simulink model "admire_sim_NDI"  (Simulink 8.4)
settings: Solver=ode4  SolverMode=SingleTasking  StartTime=0.0  StopTime=1000  FixedStep=dt  RelTol=1e-3  AbsTol=1e-6
InitFcn:
  | INIT_NDI
StartFcn:
  | tic
StopFcn:
  | toctime=toc;
  | fprintf('Actual Time = %g\nSim Time = %g\n',toctime,tout(end))
  | % Make plots
  | %admire_sim_plot
  | figure
  | plot3(yout(:,11),yout(:,10),-yout(:,12),'*-');grid
  | xlabel('East (m)');ylabel('North (m)');zlabel('Alt (m)')
  | view([0 0 1])
  | hold on
  | plot3(Ywpt,Xwpt,0*Xwpt,'r^-','MarkerSize',10)
  | axis equal
  | hold off
values from neighbouring files (symbols this model uses):
  a1 = (180*d2r)/(80^3)    (= 6.13592315154e-06)    [INIT_LINEAR.m]    (also in INIT_NDI.m)
  a2 = (24*d2r)/(80^3)    (= 8.18123086872e-07)    [INIT_LINEAR.m]    (also in INIT_NDI.m)
  Abare = [-0.0369710265542 -0.00338320638614 0 0 0.00101076287488 0 0 0 0 1.00000000002 0 1.7763568394e-12 ... (784 elements, 28x28)]    [Trim_M0p22ALT20_LinDATA.mat]    (also in Trim_M0p3ALT2000_LinDATA.mat = [-0.0208061645292 -0.00191640084378 0 0 0.000610808752105 0 )
  Altcmd_t = [ 0    1   100 200  300  425  450  550  600  700  800  880  980]    [INIT_NDI.m]
  Altcmd_v = [20  20   20   1500 1500 1500 1500 3000 3000 4000 4000 6000 6000]    [INIT_NDI.m]
  Bbare = [-1.10043807057 0.00182125944543 -0.00701366565749 0.707306131876 1.12037014439 -0.330899025785 0 0 0 0 0 0 ... (448 elements, 28x16)]    [Trim_M0p22ALT20_LinDATA.mat]    (also in Trim_M0p3ALT2000_LinDATA.mat = [-1.42042676365 -0.000549876720984 -0.00633411409606 0.84954)
  bref = 10    [INIT_NDI.m]
  C1 = ((Iy-Iz)*Iz-Ixz^2)/GG    (= -0.958151081688)    [INIT_NDI.m]
  C2 = (Ix-Iy+Iz)*Ixz/GG    (= 0.0484690861804)    [INIT_NDI.m]
  C3 = Iz/GG    (= 4.77597824802e-05)    [INIT_NDI.m]
  C4 = Ixz/GG    (= 1.18217283367e-06)    [INIT_NDI.m]
  C5 = (Iz-Ix)/Iy    (= 0.987654320988)    [INIT_NDI.m]
  C6 = Ixz/Iy    (= 0.0308641975309)    [INIT_NDI.m]
  C7 = 1/Iy    (= 1.23456790123e-05)    [INIT_NDI.m]
  C8 = (Ix*(Ix-Iy)+Ixz^2)/GG    (= -0.592859676085)    [INIT_NDI.m]
  C9 = Ix/GG    (= 9.93025180281e-06)    [INIT_NDI.m]
  CAmethod = 1    [ACA_init.m]    (also in INIT_LINEAR.m = 0; INIT_NDI.m = 0)
  Canard_max = interp1(M_vec,[25 25 25 15 15 15 15 15]*d2r,Mach,'next')    [INIT_LINEAR.m]    (also in INIT_NDI.m = [25 25 25 15 15 15 15 15]*d2r)
  Canard_min = interp1(M_vec,[-55 -55 -25 -15 -15 -15 -15 -15]*d2r,Mach,'next')    [INIT_LINEAR.m]    (also in INIT_NDI.m = [-55 -55 -25 -15 -15 -15 -15 -15]*d2r)
  CB = zeros(3,NumU)    [ACA_init.m]    (also in INIT_NDI.m = CCV*Bbare)
  CC = [C3 0 C4;0 C7 0;C4 0 C9]    [INIT_NDI.m]
  CCV = [CCV zeros(3,22)]    [INIT_LINEAR.m]    (also in INIT_NDI.m)
  cref = 5.2    [INIT_NDI.m]
  d2r = pi/180    (= 0.0174532925199)    [ACA_init.m]    (also in INIT_LINEAR.m; INIT_NDI.m)
  dalpha_err = 0    [Trim_M0p22ALT20_LinDATA.mat]    (also in Trim_M0p3ALT2000_LinDATA.mat)
  dalt_err = 0    [Trim_M0p22ALT20_LinDATA.mat]    (also in Trim_M0p3ALT2000_LinDATA.mat)
  dbeta_err = 0    [Trim_M0p22ALT20_LinDATA.mat]    (also in Trim_M0p3ALT2000_LinDATA.mat)
  ddc_bw = 0    [Trim_M0p22ALT20_LinDATA.mat]    (also in Trim_M0p3ALT2000_LinDATA.mat)
  ddc_rate = 0    [Trim_M0p22ALT20_LinDATA.mat]    (also in Trim_M0p3ALT2000_LinDATA.mat)
  ddei_bw = 0    [Trim_M0p22ALT20_LinDATA.mat]    (also in Trim_M0p3ALT2000_LinDATA.mat)
  ddei_rate = 0    [Trim_M0p22ALT20_LinDATA.mat]    (also in Trim_M0p3ALT2000_LinDATA.mat)
  ddey_bw = 0    [Trim_M0p22ALT20_LinDATA.mat]    (also in Trim_M0p3ALT2000_LinDATA.mat)
  ddey_rate = 0    [Trim_M0p22ALT20_LinDATA.mat]    (also in Trim_M0p3ALT2000_LinDATA.mat)
  ddle_bw = 0    [Trim_M0p22ALT20_LinDATA.mat]    (also in Trim_M0p3ALT2000_LinDATA.mat)
  ddle_rate = 0    [Trim_M0p22ALT20_LinDATA.mat]    (also in Trim_M0p3ALT2000_LinDATA.mat)
  ddr_bw = 0    [Trim_M0p22ALT20_LinDATA.mat]    (also in Trim_M0p3ALT2000_LinDATA.mat)
  ddr_rate = 0    [Trim_M0p22ALT20_LinDATA.mat]    (also in Trim_M0p3ALT2000_LinDATA.mat)
  dt = 0.01    [ACA_init.m]    (also in INIT_LINEAR.m; INIT_NDI.m)
  DTY_max = 0.002    [ACA_init.m]    (also in INIT_LINEAR.m; INIT_NDI.m)
  DTY_min = -0.002    [ACA_init.m]    (also in INIT_LINEAR.m; INIT_NDI.m)
  DTZ_max = 0.002    [ACA_init.m]    (also in INIT_LINEAR.m; INIT_NDI.m)
  DTZ_min = -0.002    [ACA_init.m]    (also in INIT_LINEAR.m; INIT_NDI.m)
  du = [eye(7,7)*d2r eye(7,7)*(-d2r);zeros(20,14)]    [INIT_NDI.m]
  dVt_err = 0    [Trim_M0p22ALT20_LinDATA.mat]    (also in Trim_M0p3ALT2000_LinDATA.mat)
  dx0bare = [-0.418180446269 0.000900932997672 0 0 -2.2213523116e-08 0 0 0 0 74.8477877145 0 0]    [Trim_M0p22ALT20_LinDATA.mat]    (also in Trim_M0p3ALT2000_LinDATA.mat = [-0.342751146187 0.000400431081223 0 0 -4.49007756074e-09 0 )
  Elevon_max = interp1(M_vec,[30 30 25 25 25 25 25 25]*d2r,Mach,'next')    [INIT_LINEAR.m]    (also in INIT_NDI.m = [30 30 25 25 25 25 25 25]*d2r)
  Elevon_min = interp1(M_vec,[-30 -30 -30 -30 -30 -30 -30 -30]*d2r,Mach,'next')    [INIT_LINEAR.m]    (also in INIT_NDI.m = [-30 -30 -30 -30 -30 -30 -30 -30]*d2r)
  G = [ 0 1 0 ... (first row only)    [ACA_init.m]    (also in INIT_LINEAR.m = [ 1 0 0; INIT_NDI.m)
  kcb = 2.5    [INIT_NDI.m]
  kfb = -0.4    [INIT_NDI.m]
  kib = 0.2    [INIT_NDI.m]
  kpb = 0.8    [INIT_NDI.m]
  LEF_max = interp1(M_vec,[30 30 30 20 20 15 10 10]*d2r,Mach,'next')    [INIT_LINEAR.m]    (also in INIT_NDI.m = [30 30 30 20 20 15 10 10]*d2r)
  LEF_min = interp1(M_vec,[-10 -10 -10 -10 -10 -10 -10 -10]*d2r,Mach,'next')    [INIT_LINEAR.m]    (also in INIT_NDI.m = [-10 -10 -10 -10 -10 -10 -10 -10]*d2r)
  LG_max = 1    [ACA_init.m]    (also in INIT_LINEAR.m; INIT_NDI.m)
  LG_min = 0    [ACA_init.m]    (also in INIT_LINEAR.m; INIT_NDI.m)
  LPmethod = 3    [ACA_init.m]    (also in INIT_LINEAR.m = 0; INIT_NDI.m = 0; LPwrap.m = 0; LPwrap_1.m = 0)
  M_vec = [0 0 0]    [DAwrap.m]    (also in INIT_LINEAR.m = [0 0.5 0.8 0.9 0.95 1.4 1.5 2.5]; INIT_NDI.m = [0 0.5 0.8 0.9 0.95 1.4 1.5 2.5])
  mass = 9100    [INIT_NDI.m]
  NumU = 16    [ACA_init.m]    (also in INIT_LINEAR.m; INIT_NDI.m; test.m; test_LPwrap.m)
  nwpt = 5    [INIT_NDI.m]
  PD_max = 10    [ACA_init.m]    (also in INIT_LINEAR.m; INIT_NDI.m)
  PD_min = -10    [ACA_init.m]    (also in INIT_LINEAR.m; INIT_NDI.m)
  PHIcmd_t = [0 1 1+dt 30 30+dt 60 60+dt 90 90+dt 120 120+dt 150 150+dt 180 180+dt 210 210+dt 240 240+dt 270 270+dt 300 300+dt 330 330+dt]    [INIT_NDI.m]
  PHIcmd_v = [0 0 15   15 -15   -15 0    0   30   30  -30    -30 0      0   45     45   0     0    -45   -45   0     0   -60   -60 0]    [INIT_NDI.m]
  Pmode = 3    [INIT_NDI.m]
  r2d = 180/pi    (= 57.2957795131)    [ACA_init.m]    (also in INIT_LINEAR.m; INIT_NDI.m)
  rlimit_c = 0.87260034904    [Trim_M0p22ALT20_LinDATA.mat]    (also in Trim_M0p3ALT2000_LinDATA.mat)
  rlimit_ie = 2.61780104712    [Trim_M0p22ALT20_LinDATA.mat]    (also in Trim_M0p3ALT2000_LinDATA.mat)
  rlimit_le = 0.174520069808    [Trim_M0p22ALT20_LinDATA.mat]    (also in Trim_M0p3ALT2000_LinDATA.mat)
  rlimit_oe = 2.61780104712    [Trim_M0p22ALT20_LinDATA.mat]    (also in Trim_M0p3ALT2000_LinDATA.mat)
  rlimit_r = 1.74520069808    [Trim_M0p22ALT20_LinDATA.mat]    (also in Trim_M0p3ALT2000_LinDATA.mat)
  Rmode = 3    [INIT_NDI.m]
  Rudder_max = interp1(M_vec,[30 30 25 20 15 15 15 10]*d2r,Mach,'next')    [INIT_LINEAR.m]    (also in INIT_NDI.m = [30 30 25 20 15 15 15 10]*d2r)
  Rudder_min = interp1(M_vec,[-30 -30 -25 -20 -15 -15 -15 -10]*d2r,Mach,'next')    [INIT_LINEAR.m]    (also in INIT_NDI.m = [-30 -30 -25 -20 -15 -15 -15 -10]*d2r)
  Sref = 45    [INIT_NDI.m]
  TSS_max = 1    [ACA_init.m]    (also in INIT_LINEAR.m; INIT_NDI.m)
  TSS_min = 0    [ACA_init.m]    (also in INIT_LINEAR.m; INIT_NDI.m)
  u0fcs = [0 74.8477877145 0 0 -0.0114511280235]    [Trim_M0p22ALT20_LinDATA.mat]    (also in Trim_M0p3ALT2000_LinDATA.mat = [0 99.7587452043 0 0 -0.00434812413209])
  u0new = [-0.00172441963734 -0.00172441963734 0.0557681770547 0.0557681770547 0.0557681770547 0.0557681770547 0 0 0 0.0785 0 0 ... (16 elements, 16x1)]    [Trim_M0p22ALT20_LinDATA.mat]    (also in Trim_M0p3ALT2000_LinDATA.mat = [-0.00056590748572 -0.00056590748572 0.0273345559009 0.02733)
  UD_max = 10    [ACA_init.m]    (also in INIT_LINEAR.m; INIT_NDI.m)
  UD_min = -10    [ACA_init.m]    (also in INIT_LINEAR.m; INIT_NDI.m)
  Upref = [0 0 0 0 0 0 0 0 0 0 0 0 0 0 0 0]'    [ACA_init.m]    (also in INIT_LINEAR.m; INIT_NDI.m)
  Upref_split = [[0 0 30 -30 -30 30 0]*d2r*.4 0 0 0 0 0 0 0 0 0]'    [INIT_NDI.m]
  Urlim = [350*d2r ... (first row only)    [ACA_init.m]    (also in INIT_NDI.m = [50*d2r)
  UseRL = 0    [ACA_init.m]    (also in INIT_NDI.m)
  Vcmd_t = [  0    1   100  200  300  425  450  550  600  700  800  880  980]    [INIT_NDI.m]
  Vcmd_v = Mcmd_v.*a    [INIT_NDI.m]
  VD_max = 10    [ACA_init.m]    (also in INIT_LINEAR.m; INIT_NDI.m)
  VD_min = -10    [ACA_init.m]    (also in INIT_LINEAR.m; INIT_NDI.m)
  WD_max = 10    [ACA_init.m]    (also in INIT_LINEAR.m; INIT_NDI.m)
  WD_min = -10    [ACA_init.m]    (also in INIT_LINEAR.m; INIT_NDI.m)
  Wp = W'*W    [ACA_init.m]    (also in INIT_LINEAR.m; INIT_NDI.m; test.m; test_LPwrap.m)
  Wpts = [0 1 2 3 4]    [INIT_NDI.m]
  x0 = [ max(eyp,zeros(n,1));max(-eyp,zeros(n,1));zeros(2*m,1)]    [LPwrap.m]    (also in LPwrap_1.m; LPwrap_par.m; Trim_M0p22ALT20_LinDATA.mat = [-8.62209818672e-05 -8.62209818672e-05 0.00278840885273 0.00; Trim_M0p3ALT2000_LinDATA.mat = [-2.8295374286e-05 -2.8295374286e-05 0.00136672779504 0.0013)
  x0bare = [74.8477877145 0.159877852888 0 0 0 0 0 0.159877852888 0 0 0 -20]    [Trim_M0p22ALT20_LinDATA.mat]    (also in Trim_M0p3ALT2000_LinDATA.mat = [99.7587452043 0.116024082006 0 0 0 0 0 0.116024082006 0 0 0)
  Xwpt = [0 4000 4000 0 0]*8    [INIT_NDI.m]
  y0bare = [74.8477877145 0.159877852888 0 0 0 0 0 0.159877852888 0 0 0 -20 ... (73 elements, 73x1)]    [Trim_M0p22ALT20_LinDATA.mat]    (also in Trim_M0p3ALT2000_LinDATA.mat = [99.7587452043 0.116024082006 0 0 0 0 0 0.116024082006 0 0 0)
  Ywpt = [0 0 4000 4000 0]*8    [INIT_NDI.m]
undefined symbols (not defined in the file or in its folder): CGIwrap, DAwrap, LPwrap, VJAwrap
libraries: simulink_extras x19, simulink x12
(part 2 of 5)

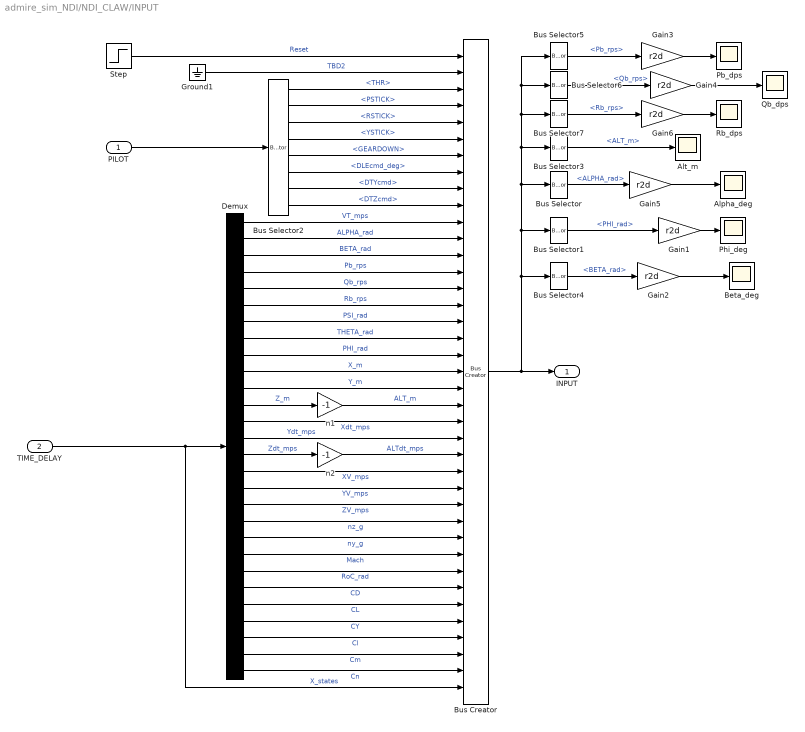
== system admire_sim_NDI/NDI_CLAW/INPUT ==
  PILOT : Inport
  TIME_DELAY : Inport  Port=2
  Alpha_deg : Scope
      settings: TimeRange=1000  YMin=0  YMax=16  SaveName=ScopeData9
  Alt_m : Scope
      settings: TimeRange=1000  YMin=0  YMax=7000  SaveName=ScopeData20
  Beta_deg : Scope
      settings: TimeRange=80  YMin=-10  YMax=15  SaveName=ScopeData32
  Bus Creator : BusCreator  Inputs=39
  Bus Selector : BusSelector  OutputSignals=ALPHA_rad
  Bus Selector1 : BusSelector  OutputSignals=PHI_rad
  Bus Selector2 : BusSelector  OutputSignals=THR,PSTICK,RSTICK,YSTICK,GEARDOWN,DLEcmd_deg,DTYcmd,DTZcmd
  Bus Selector3 : BusSelector  OutputSignals=ALT_m
  Bus Selector4 : BusSelector  OutputSignals=BETA_rad
  Bus Selector5 : BusSelector  OutputSignals=Pb_rps
  Bus Selector6 : BusSelector  OutputSignals=Qb_rps
  Bus Selector7 : BusSelector  OutputSignals=Rb_rps
  Demux : Demux  Outputs=28
  Gain{1..6} (6 alike) : Gain  Gain=r2d
  Ground1 : Ground
  Pb_dps : Scope
      settings: TimeRange=1000  YMin=-60  YMax=40  SaveName=ScopeData33
  Phi_deg : Scope
      settings: TimeRange=1000  YMin=-80  YMax=80  SaveName=ScopeData8
  Qb_dps : Scope
      settings: TimeRange=1000  YMax=10  SaveName=ScopeData34
  Rb_dps : Scope
      settings: TimeRange=80  YMin=16  YMax=22  SaveName=ScopeData35
  Step : Step  Time=dt  Before=1  After=0  SampleTime=dt
  n1 : Gain  Gain=-1
  n2 : Gain  Gain=-1
  INPUT : Outport
  wires:
  Bus Creator/1 -> INPUT/1, Bus Selector3/1, Bus Selector5/1, Bus Selector6/1, Bus Selector7/1, Bus Selector/1, Bus Selector1/1, Bus Selector4/1
  PILOT/1 -> Bus Selector2/1
  Bus Selector2/1 -> Bus Creator/3  "<THR>"
  Bus Selector2/2 -> Bus Creator/4  "<PSTICK>"
  Bus Selector2/3 -> Bus Creator/5  "<RSTICK>"
  Bus Selector2/4 -> Bus Creator/6  "<YSTICK>"
  Bus Selector2/5 -> Bus Creator/7  "<GEARDOWN>"
  Ground1/1 -> Bus Creator/2  "TBD2"
  Step/1 -> Bus Creator/1  "Reset"
  Bus Selector2/6 -> Bus Creator/8  "<DLEcmd_deg>"
  Bus Selector2/7 -> Bus Creator/9  "<DTYcmd>"
  Bus Selector2/8 -> Bus Creator/10  "<DTZcmd>"
  Demux/1 -> Bus Creator/11  "VT_mps"
  Demux/2 -> Bus Creator/12  "ALPHA_rad"
  Demux/5 -> Bus Creator/15  "Qb_rps"
  Demux/8 -> Bus Creator/18  "THETA_rad"
  Demux/3 -> Bus Creator/13  "BETA_rad"
  Demux/4 -> Bus Creator/14  "Pb_rps"
  Demux/6 -> Bus Creator/16  "Rb_rps"
  Demux/9 -> Bus Creator/19  "PHI_rad"
  Demux/10 -> Bus Creator/20  "X_m"
  Demux/11 -> Bus Creator/21  "Y_m"
  Demux/12 -> n1/1  "Z_m"
  n1/1 -> Bus Creator/22  "ALT_m"
  Demux/13 -> Bus Creator/23  "Xdt_mps"
  Demux/14 -> Bus Creator/24  "Ydt_mps"
  Demux/15 -> n2/1  "Zdt_mps"
  Demux/16 -> Bus Creator/26  "XV_mps"
  Demux/17 -> Bus Creator/27  "YV_mps"
  Demux/18 -> Bus Creator/28  "ZV_mps"
  Demux/19 -> Bus Creator/29  "nz_g"
  Demux/20 -> Bus Creator/30  "ny_g"
  Demux/21 -> Bus Creator/31  "Mach"
  Demux/22 -> Bus Creator/32  "RoC_rad"
  Demux/23 -> Bus Creator/33  "CD"
  Demux/24 -> Bus Creator/34  "CL"
  Demux/25 -> Bus Creator/35  "CY"
  Demux/26 -> Bus Creator/36  "Cl"
  Demux/27 -> Bus Creator/37  "Cm"
  Demux/28 -> Bus Creator/38  "Cn"
  Demux/7 -> Bus Creator/17  "PSI_rad"
  n2/1 -> Bus Creator/25  "ALTdt_mps"
  TIME_DELAY/1 -> Demux/1, Bus Creator/39  "X_states"
  Gain5/1 -> Alpha_deg/1
  Bus Selector/1 -> Gain5/1  "<ALPHA_rad>"
  Gain1/1 -> Phi_deg/1
  Bus Selector1/1 -> Gain1/1  "<PHI_rad>"
  Bus Selector3/1 -> Alt_m/1  "<ALT_m>"
  Gain2/1 -> Beta_deg/1
  Bus Selector4/1 -> Gain2/1  "<BETA_rad>"
  Bus Selector5/1 -> Gain3/1  "<Pb_rps>"
  Bus Selector6/1 -> Gain4/1  "<Qb_rps>"
  Bus Selector7/1 -> Gain6/1  "<Rb_rps>"
  Gain3/1 -> Pb_dps/1
  Gain4/1 -> Qb_dps/1
  Gain6/1 -> Rb_dps/1

== system admire_sim_NDI/NDI_CLAW/MissionManager ==
  INPUT : Inport
  ALT_table : Lookup  InputValues=Altcmd_t  Table=Altcmd_v  LookUpMeth=Interpolation-Use End Values
  Bus Creator : BusCreator  Inputs=8
  Bus Selector3 : BusSelector  OutputSignals=Xcmd,Xcmdm1,Ycmd,Ycmdm1,PHImax_rad
  Constant : Constant  Value=Vcmd_v(1)
  Constant1 : Constant  Value=Altcmd_v(1)
  Constant2 : Constant  Value=x0bare(1)
  Constant3 : Constant  Value=-x0bare(12)+50
  Constant4 : Constant  Value=-120
  Digital Clock : DigitalClock  SampleTime=dt
  Gain : Gain  Gain=0
  PHI_5 : Lookup  InputValues=PHIcmd_t  Table=PHIcmd_v  LookUpMeth=Interpolation-Use End Values
  Saturation : Saturate  UpperLimit=300  LowerLimit=0
  Sum : Sum  Inputs=|++
  V_table : Lookup  InputValues=Vcmd_t  Table=Vcmd_v  LookUpMeth=Interpolation-Use End Values
  WaypointNavigation : Subsystem
  MM : Outport
  wires:
  Digital Clock/1 -> Sum/1, V_table/1, ALT_table/1
  Bus Creator/1 -> MM/1
  PHI_5/1 -> Bus Creator/3  "PHIcmd_deg"
  INPUT/1 -> WaypointNavigation/1(INPUT)
  WaypointNavigation/1(WN) -> Bus Selector3/1
  Bus Selector3/1 -> Bus Creator/4  "<Xcmd>"
  Bus Selector3/2 -> Bus Creator/5  "<Xcmdm1>"
  Bus Selector3/3 -> Bus Creator/6  "<Ycmd>"
  Bus Selector3/4 -> Bus Creator/7  "<Ycmdm1>"
  Bus Selector3/5 -> Bus Creator/8  "<PHImax_rad>"
  V_table/1 -> Bus Creator/2  "Vcmd_mps"
  ALT_table/1 -> Bus Creator/1  "ALTcmd_m"
  Sum/1 -> Saturation/1
  Constant4/1 -> Sum/2
  Saturation/1 -> Gain/1
  Gain/1 -> PHI_5/1

== system admire_sim_NDI/NDI_CLAW/PILOT_Mod ==
  In1 : Inport
  Bus Creator1 : BusCreator  Inputs=9
  Bus Selector : BusSelector  OutputSignals=Fes_out,Vt_out,Fas_out,Frp_out,dle_out,ldg_out,dty_out,dtz_out,tss_out
  Gain1 : Gain  Gain=1/80
  Gain{2,5..9} (6 alike) : Gain
  Gain3 : Gain  Gain=1/80
  Gain4 : Gain  Gain=1/200
  PILOT : Outport
  wires:
  In1/1 -> Bus Selector/1
  Bus Selector/1 -> Gain1/1  "<Fes_out>"
  Bus Selector/2 -> Gain2/1  "<Vt_out>"
  Bus Selector/3 -> Gain3/1  "<Fas_out>"
  Bus Selector/4 -> Gain4/1  "<Frp_out>"
  Bus Selector/5 -> Gain5/1  "<dle_out>"
  Bus Selector/6 -> Gain6/1  "<ldg_out>"
  Bus Selector/7 -> Gain7/1  "<dty_out>"
  Bus Selector/8 -> Gain8/1  "<dtz_out>"
  Gain1/1 -> Bus Creator1/1  "PSTICK"
  Gain2/1 -> Bus Creator1/2  "Vcmd_mps"
  Gain3/1 -> Bus Creator1/3  "RSTICK"
  Gain4/1 -> Bus Creator1/4  "YSTICK"
  Gain5/1 -> Bus Creator1/5  "DLEcmd_deg"
  Gain6/1 -> Bus Creator1/6  "GEARDOWN"
  Gain7/1 -> Bus Creator1/7  "DTYcmd"
  Gain8/1 -> Bus Creator1/8  "DTZcmd"
  Gain9/1 -> Bus Creator1/9  "THR"
  Bus Creator1/1 -> PILOT/1
  Bus Selector/9 -> Gain9/1  "<tss_out>"

== system admire_sim_NDI/PILOT/Doublet ==
  Gain : Gain  Gain=.1
  Step : Step  SampleTime=0
  Step1 : Step  Time=1.1  After=-2  SampleTime=0
  Step2 : Step  Time=1.2  SampleTime=0
  Sum8 : Sum  Inputs=+++
  Out1 : Outport
  wires:
  Step/1 -> Sum8/1
  Step1/1 -> Sum8/2
  Step2/1 -> Sum8/3
  Sum8/1 -> Gain/1
  Gain/1 -> Out1/1

== system admire_sim_NDI/Aircraft response1/Sensor models/Subsystem To Gain-Scheduling ==
  note: Level III
  Vt [m/s] : Inport
  alt [m] : Inport  Port=2
  S-Function : S-Function  FunctionName=machno  EnableBusSupport=off
  Mach : Outport
  tag scope: Altitude=global, Mach=global
  wires:
  alt [m]/1 -> [Altitude], S-Function/2
  Vt [m/s]/1 -> S-Function/1
  S-Function/1 -> [Mach], Mach/1

== system admire_sim_NDI/NDI_CLAW/DynamicInversionControl/AERO_OBM ==
  INPUT : Inport
  uz : Inport  Port=2
  AeroLimits : Subsystem
  Bus Creator1 : BusCreator  Inputs=5
  Bus Selector : BusSelector  OutputSignals=Unom
  LinearOBM : Subsystem
  NonLinearOBM : Subsystem
  OBM : Outport
  wires:
  AeroLimits/1(Umin) -> Bus Creator1/4
  AeroLimits/2(Umax) -> Bus Creator1/5
  Bus Creator1/1 -> OBM/1
  uz/1 -> LinearOBM/2(uz), Bus Selector/1, NonLinearOBM/2(uz)
  Bus Selector/1 -> Bus Creator1/3  "<Unom>"
  INPUT/1 -> LinearOBM/1(INPUT), AeroLimits/1(Input), NonLinearOBM/1(INPUT)
  NonLinearOBM/1(CVdt_nom) -> Bus Creator1/1
  NonLinearOBM/2(CB) -> Bus Creator1/2

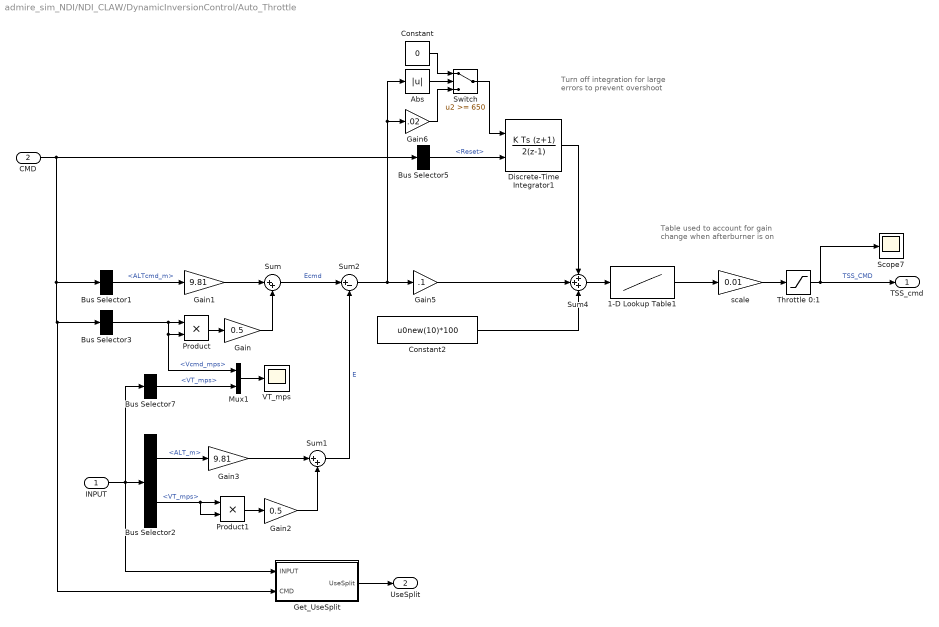
== system admire_sim_NDI/NDI_CLAW/DynamicInversionControl/Auto_Throttle ==
  note: Turn off integration for large
      | errors to prevent overshoot
  note: Table used to account for gain
      | change when afterburner is on
  INPUT : Inport
  CMD : Inport  Port=2
  1-D Lookup Table1 : Lookup_n-D  NumberOfTableDimensions=1  BreakpointsForDimension1=[0 80 300]  Table=[0 80 100]  ExtrapMethod=Clip  UseLastTableValue=on  RndMeth=Simplest  InputSameDT=on
  Abs : Abs
  Bus Selector1 : BusSelector  OutputSignals=ALTcmd_m
  Bus Selector2 : BusSelector  OutputSignals=ALT_m,VT_mps
  Bus Selector3 : BusSelector  OutputSignals=Vcmd_mps
  Bus Selector5 : BusSelector  OutputSignals=Reset
  Bus Selector7 : BusSelector  OutputSignals=VT_mps
  Constant : Constant  Value=0
  Constant2 : Constant  Value=u0new(10)*100
  Discrete-Time Integrator1 : DiscreteIntegrator  IntegratorMethod=Integration: Trapezoidal  ExternalReset=level  SampleTime=dt  LimitOutput=on  LowerSaturationLimit=-50
  Gain : Gain  Gain=0.5
  Gain1 : Gain  Gain=9.81
  Gain2 : Gain  Gain=0.5
  Gain3 : Gain  Gain=9.81
  Gain5 : Gain  Gain=.1
  Gain6 : Gain  Gain=.02
  Get_UseSplit : Subsystem
  Mux1 : Mux  Inputs=2
  Product : Product  RndMeth=Zero
  Product1 : Product  RndMeth=Zero
  Scope7 : Scope
      settings: TimeRange=20  YMin=0  YMax=1  SaveName=ScopeData11
  Sum : Sum  Inputs=|++
  Sum1 : Sum  Inputs=|++
  Sum2 : Sum  Inputs=|+-
  Sum4 : Sum  Inputs=+++
  Switch : Switch  Threshold=650
  Throttle 0:1 : Saturate  UpperLimit=TSS_max  LowerLimit=TSS_min  RndMeth=Ceiling
  VT_mps : Scope
      settings: TimeRange=1000  YMin=50  YMax=450  SaveName=ScopeData58
  scale : Gain  Gain=0.01
  TSS_cmd : Outport
  UseSplit : Outport  Port=2
  wires:
  CMD/1 -> Bus Selector1/1, Get_UseSplit/2(CMD), Bus Selector3/1, Bus Selector5/1
  Product/1 -> Gain/1
  Gain/1 -> Sum/2
  Product1/1 -> Gain2/1
  Bus Selector2/1 -> Gain3/1  "<ALT_m>"
  Gain2/1 -> Sum1/2
  Bus Selector2/2 -> Product1/1, Product1/2  "<VT_mps>"
  Sum/1 -> Sum2/1  "Ecmd"
  Sum1/1 -> Sum2/2  "E"
  Bus Selector5/1 -> Discrete-Time Integrator1/2  "<Reset>"
  Discrete-Time Integrator1/1 -> Sum4/1
  Sum2/1 -> Gain5/1, Gain6/1, Abs/1
  Bus Selector1/1 -> Gain1/1  "<ALTcmd_m>"
  Bus Selector3/1 -> Product/1, Product/2, Mux1/1  "<Vcmd_mps>"
  Sum4/1 -> 1-D Lookup Table1/1
  Abs/1 -> Switch/2
  Switch/1 -> Discrete-Time Integrator1/1
  Constant/1 -> Switch/1
  Gain6/1 -> Switch/3
  INPUT/1 -> Get_UseSplit/1(INPUT), Bus Selector7/1, Bus Selector2/1
  1-D Lookup Table1/1 -> scale/1
  Gain5/1 -> Sum4/2
  Mux1/1 -> VT_mps/1
  Bus Selector7/1 -> Mux1/2  "<VT_mps>"
  Get_UseSplit/1(UseSplit) -> UseSplit/1
  Constant2/1 -> Sum4/3
  scale/1 -> Throttle 0:1/1
  Throttle 0:1/1 -> TSS_cmd/1, Scope7/1  "TSS_CMD"
  Gain1/1 -> Sum/1
  Gain3/1 -> Sum1/1

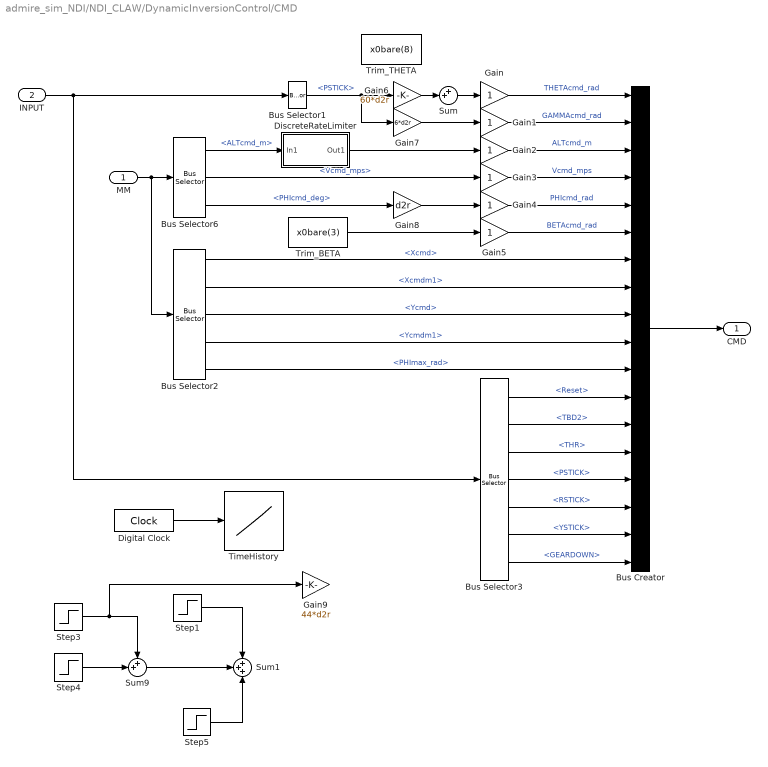
== system admire_sim_NDI/NDI_CLAW/DynamicInversionControl/CMD ==
  MM : Inport
  INPUT : Inport  Port=2
  Bus Creator : BusCreator  Inputs=18
  Bus Selector1 : BusSelector  OutputSignals=PSTICK
  Bus Selector2 : BusSelector  OutputSignals=Xcmd,Xcmdm1,Ycmd,Ycmdm1,PHImax_rad
  Bus Selector3 : BusSelector  OutputSignals=Reset,TBD2,THR,PSTICK,RSTICK,YSTICK,GEARDOWN
  Bus Selector6 : BusSelector  OutputSignals=ALTcmd_m,Vcmd_mps,PHIcmd_deg
  Digital Clock : DigitalClock  SampleTime=dt
  DiscreteRateLimiter : Subsystem
  Gain{,1..5} (6 alike) : Gain
  Gain6 : Gain  Gain=60*d2r
  Gain7 : Gain  Gain=6*d2r
  Gain8 : Gain  Gain=d2r
  Gain9 : Gain  Gain=44*d2r
  Step1 : Step  Time=70  SampleTime=dt
  Step3 : Step  Time=50  SampleTime=dt
  Step4 : Step  Time=60  After=-1  SampleTime=dt
  Step5 : Step  Time=60  After=-1  SampleTime=dt
  Sum : Sum  Inputs=++|
  Sum1 : Sum  Inputs=+++
  Sum9 : Sum  Inputs=++|
  TimeHistory : Lookup  InputValues=[0 20 30 40 50 60]  Table=[0 0 3 3 0 0]*d2r  LookUpMeth=Interpolation-Use End Values
  Trim_BETA : Constant  Value=x0bare(3)
  Trim_THETA : Constant  Value=x0bare(8)
  CMD : Outport
  wires:
  Bus Creator/1 -> CMD/1
  Gain/1 -> Bus Creator/1  "THETAcmd_rad"
  Gain1/1 -> Bus Creator/2  "GAMMAcmd_rad"
  Gain2/1 -> Bus Creator/3  "ALTcmd_m"
  Gain3/1 -> Bus Creator/4  "Vcmd_mps"
  Gain4/1 -> Bus Creator/5  "PHIcmd_rad"
  Gain5/1 -> Bus Creator/6  "BETAcmd_rad"
  Bus Selector1/1 -> Gain6/1, Gain7/1  "<PSTICK>"
  INPUT/1 -> Bus Selector1/1, Bus Selector3/1
  Gain7/1 -> Gain1/1
  Gain6/1 -> Sum/2
  Sum/1 -> Gain/1
  MM/1 -> Bus Selector6/1, Bus Selector2/1
  Bus Selector6/1 -> DiscreteRateLimiter/1(In1)  "<ALTcmd_m>"
  Bus Selector6/2 -> Gain3/1  "<Vcmd_mps>"
  Bus Selector6/3 -> Gain8/1  "<PHIcmd_deg>"
  Bus Selector2/1 -> Bus Creator/7  "<Xcmd>"
  Bus Selector2/2 -> Bus Creator/8  "<Xcmdm1>"
  Bus Selector2/3 -> Bus Creator/9  "<Ycmd>"
  Bus Selector2/4 -> Bus Creator/10  "<Ycmdm1>"
  Bus Selector2/5 -> Bus Creator/11  "<PHImax_rad>"
  Bus Selector3/1 -> Bus Creator/12  "<Reset>"
  Bus Selector3/2 -> Bus Creator/13  "<TBD2>"
  Bus Selector3/3 -> Bus Creator/14  "<THR>"
  Bus Selector3/4 -> Bus Creator/15  "<PSTICK>"
  Bus Selector3/5 -> Bus Creator/16  "<RSTICK>"
  Bus Selector3/6 -> Bus Creator/17  "<YSTICK>"
  Bus Selector3/7 -> Bus Creator/18  "<GEARDOWN>"
  Step3/1 -> Sum9/1, Gain9/1
  Step4/1 -> Sum9/2
  Sum9/1 -> Sum1/2
  Step1/1 -> Sum1/1
  Digital Clock/1 -> TimeHistory/1
  Step5/1 -> Sum1/3
  Trim_BETA/1 -> Gain5/1
  DiscreteRateLimiter/1(Out1) -> Gain2/1
  Gain8/1 -> Gain4/1

== system admire_sim_NDI/NDI_CLAW/DynamicInversionControl/ControlAllocation ==
  TSS_cmd : Inport
  UseSplit : Inport  Port=2
  CVdt_des : Inport  Port=3
  OBM : Inport  Port=4
  GetU : Subsystem
  PostProcess : Subsystem
  PreProcess : Subsystem
  Ucmd : Outport
  wires:
  PreProcess/1(PrePro) -> GetU/1(PrePro), PostProcess/2(PrePro)
  GetU/1(u) -> PostProcess/1(u)
  CVdt_des/1 -> PreProcess/1(CVdt_des)  "CVdt_des"
  OBM/1 -> PreProcess/2(OBM)
  UseSplit/1 -> PostProcess/3(UseSplit)
  PostProcess/1(Ucmd) -> Ucmd/1
  TSS_cmd/1 -> PostProcess/4(TSS_cmd)

== system admire_sim_NDI/NDI_CLAW/DynamicInversionControl/REG ==
  CMD : Inport
  INPUT : Inport  Port=2
  Mux : Mux  Inputs=3
  PitchReg : Subsystem
  RollReg : Subsystem
  YawReg : Subsystem
  CVdt_des : Outport
  wires:
  CMD/1 -> RollReg/1(CMD), YawReg/1(CMD), PitchReg/1(CMD)
  Mux/1 -> CVdt_des/1  "CVdt_des"
  PitchReg/1(MCVdt) -> Mux/2
  RollReg/1(LCVdt) -> Mux/1
  YawReg/1(NCVdt) -> Mux/3
  INPUT/1 -> RollReg/2(INPUT), PitchReg/2(INPUT), YawReg/2(INPUT)

== system admire_sim_NDI/NDI_CLAW/DynamicInversionControl/UcmdScope ==
  In1 : Inport
  Demux : Demux  Outputs=7
  Selector : Selector  InputPortWidth=16  Indices=[1:7]
  Ucmd_deg : Scope  NumInputPorts=7
      settings: TimeRange=1000  YMin=-10~-10~-10~-20~-20~-10~-4  YMax=10~10~20~10~10~20~4  SaveName=ScopeData51
  scale1 : Gain  Gain=r2d
  wires:
  Selector/1 -> scale1/1
  scale1/1 -> Demux/1
  In1/1 -> Selector/1
  Demux/2 -> Ucmd_deg/2  "LC_deg"
  Demux/1 -> Ucmd_deg/1  "RC_deg"
  Demux/5 -> Ucmd_deg/5  "LIE_deg"
  Demux/7 -> Ucmd_deg/7  "RUD_deg"
  Demux/6 -> Ucmd_deg/6  "LOE_deg"
  Demux/3 -> Ucmd_deg/3  "ROE_deg"
  Demux/4 -> Ucmd_deg/4  "RIE_deg"

== system admire_sim_NDI/NDI_CLAW/DynamicInversionControl/Unom ==
  Ucmd : Inport
  Bus Creator : BusCreator  Inputs=2
  Discrete-Time Integrator : DiscreteIntegrator  IntegratorMethod=Integration: Trapezoidal  InitialCondition=u0new  SampleTime=dt
  Get_Unom : Subsystem
  Sum2 : Sum  Inputs=|+-
  Unit Delay1 : UnitDelay  InitialCondition=u0new  SampleTime=dt
  Unit Delay2 : UnitDelay  InitialCondition=u0new  SampleTime=dt
  scale1 : Gain
  scale2 : Gain  Gain=20
  Upast : Outport
  wires:
  Discrete-Time Integrator/1 -> Unit Delay2/1, scale1/1
  Unit Delay1/1 -> Sum2/1, Get_Unom/2(Uz)
  Sum2/1 -> scale2/1
  Unit Delay2/1 -> Sum2/2
  scale2/1 -> Discrete-Time Integrator/1
  Ucmd/1 -> Unit Delay1/1
  scale1/1 -> Get_Unom/1(Uact), Bus Creator/1  "Uact"
  Get_Unom/1(Unom) -> Bus Creator/2
  Bus Creator/1 -> Upast/1

== system admire_sim_NDI/NDI_CLAW/MissionManager/WaypointNavigation ==
  INPUT : Inport
  Bus Creator1 : BusCreator  Inputs=7
  Bus Creator2 : BusCreator  Inputs=6
  Bus Selector : BusSelector  OutputSignals=npt
  Bus Selector1 : BusSelector  OutputSignals=npt
  Bus Selector2 : BusSelector  OutputSignals=nptm1
  Bus Selector3 : BusSelector  OutputSignals=nptm1
  Bus Selector4 : BusSelector  OutputSignals=nptp1
  Bus Selector5 : BusSelector  OutputSignals=nptp1
  Bus Selector6 : BusSelector  OutputSignals=Xcmd,Xcmdm1,Xcmdp1,Ycmd,Ycmdm1,Ycmdp1  OutputAsBus=on
  ChangeWptNumber : Subsystem
  Demux : Demux  Outputs=6
  GetWptNumber : Subsystem
  Unit Delay : UnitDelay  SampleTime=dt
  Xcmd : Lookup_n-D  NumberOfTableDimensions=1  BreakpointsForDimension1=Wpts  Table=Xwpt  InterpMethod=Flat  OutDataTypeStr=double  RndMeth=Simplest  InputSameDT=on
  Xcmdm1 : Lookup_n-D  NumberOfTableDimensions=1  BreakpointsForDimension1=Wpts  Table=Xwpt  InterpMethod=Flat  OutDataTypeStr=double  RndMeth=Simplest  InputSameDT=on
  Xcmdp1 : Lookup_n-D  NumberOfTableDimensions=1  BreakpointsForDimension1=Wpts  Table=Xwpt  InterpMethod=Flat  OutDataTypeStr=double  RndMeth=Simplest  InputSameDT=on
  Ycmd : Lookup_n-D  NumberOfTableDimensions=1  BreakpointsForDimension1=Wpts  Table=Ywpt  InterpMethod=Flat  OutDataTypeStr=double  RndMeth=Simplest  InputSameDT=on
  Ycmdm1 : Lookup_n-D  NumberOfTableDimensions=1  BreakpointsForDimension1=Wpts  Table=Ywpt  InterpMethod=Flat  OutDataTypeStr=double  RndMeth=Simplest  InputSameDT=on
  Ycmdp11 : Lookup_n-D  NumberOfTableDimensions=1  BreakpointsForDimension1=Wpts  Table=Ywpt  InterpMethod=Flat  OutDataTypeStr=double  RndMeth=Simplest  InputSameDT=on
  WN : Outport
  wires:
  Bus Selector/1 -> Xcmd/1  "<npt>"
  Bus Selector1/1 -> Ycmd/1  "<npt>"
  Bus Selector2/1 -> Xcmdm1/1  "<nptm1>"
  Bus Selector3/1 -> Ycmdm1/1  "<nptm1>"
  Xcmd/1 -> Bus Creator1/1  "Xcmd"
  Xcmdm1/1 -> Bus Creator1/2  "Xcmdm1"
  Bus Creator1/1 -> Bus Selector6/1, WN/1
  INPUT/1 -> ChangeWptNumber/1(INPUT)
  ChangeWptNumber/1(NextPt) -> GetWptNumber/1(NextPt)
  Unit Delay/1 -> Demux/1
  Demux/1 -> Bus Creator2/1  "Xcmd"
  Demux/2 -> Bus Creator2/2  "Xcmdm1"
  Demux/3 -> Bus Creator2/3  "Xcmdp1"
  Demux/4 -> Bus Creator2/4  "Ycmd"
  Bus Creator2/1 -> ChangeWptNumber/2(WNz)
  Bus Selector4/1 -> Xcmdp1/1  "<nptp1>"
  Bus Selector5/1 -> Ycmdp11/1  "<nptp1>"
  GetWptNumber/1(Out1) -> Bus Selector/1, Bus Selector2/1, Bus Selector4/1, Bus Selector3/1, Bus Selector5/1, Bus Selector1/1
  Xcmdp1/1 -> Bus Creator1/3  "Xcmdp1"
  Ycmd/1 -> Bus Creator1/4  "Ycmd"
  Ycmdm1/1 -> Bus Creator1/5  "Ycmdm1"
  Ycmdp11/1 -> Bus Creator1/6  "Ycmdp1"
  Demux/5 -> Bus Creator2/5  "Ycmdm1"
  Demux/6 -> Bus Creator2/6  "Ycmdp1"
  Bus Selector6/1 -> Unit Delay/1
  ChangeWptNumber/2(PHImax_rad) -> Bus Creator1/7

== system admire_sim_NDI/NDI_CLAW/DynamicInversionControl/AERO_OBM/AeroLimits ==
  Input : Inport
  Bus Selector1 : BusSelector  OutputSignals=Mach
  Get_Umax : Subsystem
  Get_Umin : Subsystem
  Umin : Outport
  Umax : Outport  Port=2
  wires:
  Bus Selector1/1 -> Get_Umax/1(Mach), Get_Umin/1(Mach)  "<Mach>"
  Input/1 -> Bus Selector1/1
  Get_Umin/1(Umin) -> Umin/1
  Get_Umax/1(Umax) -> Umax/1

== system admire_sim_NDI/NDI_CLAW/DynamicInversionControl/AERO_OBM/LinearOBM ==
  INPUT : Inport
  uz : Inport  Port=2
  B : Gain  Gain=Bbare  Multiplication=Matrix(K*u)
  Bus Selector : BusSelector  OutputSignals=Unom
  Bus Selector2 : BusSelector  OutputSignals=X_states
  CA : Gain  Gain=Abare  Multiplication=Matrix(K*u)
  CB_const : Constant  Value=CB
  CCV : Gain  Gain=CCV  Multiplication=Matrix(K*u)
  Sum : Sum  Inputs=|+-
  Sum2 : Sum  Inputs=|++
  Trim_x : Constant  Value=[x0bare;zeros(16,1)]
  CVdt_nom : Outport
  CB : Outport  Port=2
  wires:
  Bus Selector2/1 -> Sum/1  "<X_states>"
  Sum/1 -> CA/1
  Trim_x/1 -> Sum/2
  CA/1 -> Sum2/1
  Sum2/1 -> CCV/1
  B/1 -> Sum2/2
  INPUT/1 -> Bus Selector2/1
  CCV/1 -> CVdt_nom/1  "CVdt_nom"
  CB_const/1 -> CB/1  "CB"
  Bus Selector/1 -> B/1  "<Unom>"
  uz/1 -> Bus Selector/1

== system admire_sim_NDI/NDI_CLAW/DynamicInversionControl/AERO_OBM/NonLinearOBM ==
  INPUT : Inport
  uz : Inport  Port=2
  Bus Selector3 : BusSelector  OutputSignals=X_states
  Constant : Constant  Value=CB(:,8:16)
  Get_B_Aero : Subsystem
  Get_u0 : Subsystem
  Matrix Concatenate : Concatenate  Mode=Multidimensional array  ConcatenateDimension=2
  CVdt_nom : Outport
  CB : Outport  Port=2
  wires:
  Bus Selector3/1 -> Get_B_Aero/1(Sensors)  "<X_states>"
  Get_u0/1(u0) -> Get_B_Aero/2(u0)
  Get_B_Aero/2(B) -> Matrix Concatenate/1
  Get_B_Aero/1(CVdt) -> CVdt_nom/1  "CVdt_nom"
  INPUT/1 -> Bus Selector3/1, Get_u0/1(INPUT)
  uz/1 -> Get_B_Aero/3(uz), Get_u0/2(uz)
  Constant/1 -> Matrix Concatenate/2
  Matrix Concatenate/1 -> CB/1  "CB"

== system admire_sim_NDI/NDI_CLAW/DynamicInversionControl/Auto_Throttle/Get_UseSplit ==
  note: UseSplit is true when you want to use
      | the wing trailing edge effectors to act as a
      | speedbrake.  This is done by biasing the
      | inboard surfaces up and the outboard surfaces down.
  note: NOTE: Velocity commands should ramp, not step, for this to work
  INPUT : Inport
  CMD : Inport  Port=2
  Bus Selector4 : BusSelector  OutputSignals=Vcmd_mps
  Bus Selector6 : BusSelector  OutputSignals=Mach
  Compare To Constant : simulink/Logic and Bit Operations/Compare To Constant  SystemSampleTime=-1  relop=<=  const=-0.007  LogicOutDataTypeMode=uint8
  Compare To Constant1 : simulink/Logic and Bit Operations/Compare To Constant  SystemSampleTime=-1  relop=>=  const=0.3  LogicOutDataTypeMode=uint8
  Compare To Constant3 : simulink/Logic and Bit Operations/Compare To Constant  SystemSampleTime=-1  relop=<=  const=0.8  LogicOutDataTypeMode=uint8
  Logical Operator : Logic  AllPortsSameDT=off  OutDataTypeStr=boolean
  Logical Operator1 : Logic  AllPortsSameDT=off  OutDataTypeStr=boolean
  Sum5 : Sum  Inputs=|-+
  Unit Delay : UnitDelay  SampleTime=dt
  UseSplit : Outport
  wires:
  CMD/1 -> Bus Selector4/1
  Bus Selector6/1 -> Compare To Constant3/1, Compare To Constant1/1  "<Mach>"
  Bus Selector4/1 -> Sum5/2, Unit Delay/1  "<Vcmd_mps>"
  Sum5/1 -> Compare To Constant/1
  Logical Operator/1 -> UseSplit/1
  Compare To Constant1/1 -> Logical Operator1/1
  Logical Operator1/1 -> Logical Operator/1
  Compare To Constant3/1 -> Logical Operator1/2
  Compare To Constant/1 -> Logical Operator/2
  Unit Delay/1 -> Sum5/1
  INPUT/1 -> Bus Selector6/1

== system admire_sim_NDI/NDI_CLAW/DynamicInversionControl/CMD/DiscreteRateLimiter ==
  In1 : Inport
  Saturation1 : Saturate  UpperLimit=20*dt  LowerLimit=-15*dt
  Sum5 : Sum  Inputs=|+-
  Sum6 : Sum  Inputs=|++
  Unit Delay : UnitDelay  InitialCondition=-x0bare(12)  SampleTime=dt
  Out1 : Outport
  wires:
  Sum5/1 -> Saturation1/1
  Saturation1/1 -> Sum6/1
  In1/1 -> Sum5/1
  Sum6/1 -> Out1/1, Unit Delay/1
  Unit Delay/1 -> Sum6/2, Sum5/2

== system admire_sim_NDI/NDI_CLAW/DynamicInversionControl/ControlAllocation/GetU ==
  PrePro : Inport
  CAmethod : Constant  Value=CAmethod  OutDataTypeStr=int8
  CGI_4 : Subsystem  TreatAsAtomicUnit=on
  DirectAllocation_3 : Subsystem  TreatAsAtomicUnit=on
  If : If  IfExpression=u1 == 0  ElseIfExpressions=u1 ==1, u1==2, u1==3, u1==4, u1==5
  LP_6 : Subsystem  TreatAsAtomicUnit=on
  MakeINMAT : Subsystem
  MakeSquare_0 : Subsystem  TreatAsAtomicUnit=on
  Merge : Merge  Inputs=7
  VJA_5 : Subsystem  TreatAsAtomicUnit=on
  WeightedPseudo Clipped_1 : Subsystem  TreatAsAtomicUnit=on
  WeightedPseudo Scaled_2 : Subsystem  TreatAsAtomicUnit=on
  u : Outport
  wires:
  CAmethod/1 -> If/1
  If/1 -> MakeSquare_0/Action
  If/2 -> WeightedPseudo Clipped_1/Action
  If/3 -> WeightedPseudo Scaled_2/Action
  If/4 -> DirectAllocation_3/Action
  VJA_5/1(Out1) -> Merge/2
  MakeSquare_0/1(Out1) -> Merge/7
  WeightedPseudo Clipped_1/1(Out1) -> Merge/6
  WeightedPseudo Scaled_2/1(Out1) -> Merge/5
  DirectAllocation_3/1(Out1) -> Merge/4
  If/5 -> CGI_4/Action
  CGI_4/1(Out1) -> Merge/3
  If/6 -> VJA_5/Action
  Merge/1 -> u/1
  If/7 -> LP_6/Action
  LP_6/1(Out1) -> Merge/1
  PrePro/1 -> MakeINMAT/1(In1), DirectAllocation_3/1(In1), WeightedPseudo Scaled_2/1(In1), WeightedPseudo Clipped_1/1(In1), MakeSquare_0/1(In1)
  MakeINMAT/1(Out1) -> LP_6/1(In1), VJA_5/1(In1), CGI_4/1(In1)

== system admire_sim_NDI/NDI_CLAW/DynamicInversionControl/ControlAllocation/PostProcess ==
  u : Inport
  PrePro : Inport  Port=2
  UseSplit : Inport  Port=3
  TSS_cmd : Inport  Port=4
  Bus Selector1 : BusSelector  OutputSignals=Unom
  DriveToPreferred : Subsystem
  Subsystem : Subsystem
  Sum2 : Sum  Inputs=|++
  Sum3 : Sum  Inputs=|++
  Ucmd : Outport
  wires:
  Sum2/1 -> Sum3/1
  Sum3/1 -> Subsystem/1(In1)
  u/1 -> DriveToPreferred/2(u), Sum2/1
  PrePro/1 -> DriveToPreferred/1(PrePro), Bus Selector1/1
  UseSplit/1 -> DriveToPreferred/3(UseSplit)
  TSS_cmd/1 -> Subsystem/2(TSS_cmd)
  Subsystem/1(Ucmd) -> Ucmd/1
  Bus Selector1/1 -> Sum2/2  "<Unom>"
  DriveToPreferred/1(Out2) -> Sum3/2

== system admire_sim_NDI/NDI_CLAW/DynamicInversionControl/ControlAllocation/PreProcess ==
  CVdt_des : Inport
  OBM : Inport  Port=2
  Bus Creator : BusCreator  Inputs=6
  Bus Selector : BusSelector  OutputSignals=CB
  Bus Selector2 : BusSelector  OutputSignals=Unom
  Constant : Constant  Value=[1 1 1 1 1 1 1 0 0 0 0 0 0 0 0 0]
  GetLimits : Subsystem
  PrePro : Outport
  wires:
  CVdt_des/1 -> Bus Creator/1
  OBM/1 -> Bus Selector/1, Bus Selector2/1, GetLimits/1(OBM)
  Bus Selector/1 -> Bus Creator/2  "<CB>"
  Bus Creator/1 -> PrePro/1
  Bus Selector2/1 -> Bus Creator/3  "<Unom>"
  GetLimits/1(Umin) -> Bus Creator/4
  GetLimits/2(Umax) -> Bus Creator/5
  Constant/1 -> Bus Creator/6  "INDX"

== system admire_sim_NDI/NDI_CLAW/DynamicInversionControl/REG/PitchReg ==
  CMD : Inport
  INPUT : Inport  Port=2
  ALTCMD_3 : Subsystem
  GAMMACMD_2 : Subsystem
  If : If  IfExpression=u1 ==1  ElseIfExpressions=u1 == 2  SampleTime=dt
  Merge : Merge  Inputs=3
  Pmode : Constant  Value=Pmode  OutDataTypeStr=int8
  QCMD_1 : Subsystem
  MCVdt : Outport
  wires:
  Merge/1 -> MCVdt/1
  CMD/1 -> ALTCMD_3/1(CMD), QCMD_1/1(CMD), GAMMACMD_2/1(CMD)
  If/3 -> ALTCMD_3/Action
  If/2 -> GAMMACMD_2/Action
  If/1 -> QCMD_1/Action
  ALTCMD_3/1(MCVdt) -> Merge/1
  GAMMACMD_2/1(MCVdt) -> Merge/2
  QCMD_1/1(MCVdt) -> Merge/3
  INPUT/1 -> ALTCMD_3/2(INPUT), GAMMACMD_2/2(INPUT), QCMD_1/2(INPUT)
  Pmode/1 -> If/1

== system admire_sim_NDI/NDI_CLAW/DynamicInversionControl/REG/RollReg ==
  CMD : Inport
  INPUT : Inport  Port=2
  If : If  IfExpression=u1 ==1  ElseIfExpressions=u1 == 2  SampleTime=dt
  Merge : Merge  Inputs=3
  PHIcmd_2 : Subsystem
  Pcmd_1 : Subsystem
  Rmode : Constant  Value=Rmode  OutDataTypeStr=int8
  XTKcmd_3 : Subsystem
  LCVdt : Outport
  wires:
  CMD/1 -> XTKcmd_3/1(CMD), Pcmd_1/1(CMD), PHIcmd_2/1(CMD)
  If/1 -> Pcmd_1/Action
  If/2 -> PHIcmd_2/Action
  If/3 -> XTKcmd_3/Action
  XTKcmd_3/1(LCVdt) -> Merge/1
  PHIcmd_2/1(LCVdt) -> Merge/2
  Pcmd_1/1(LCVdt) -> Merge/3
  Merge/1 -> LCVdt/1
  INPUT/1 -> XTKcmd_3/2(INPUT), PHIcmd_2/2(INPUT), Pcmd_1/2(INPUT)
  Rmode/1 -> If/1

== system admire_sim_NDI/NDI_CLAW/DynamicInversionControl/REG/YawReg ==
  CMD : Inport
  INPUT : Inport  Port=2
  Bus Selector1 : BusSelector  OutputSignals=BETA_rad
  Bus Selector3 : BusSelector  OutputSignals=BETAcmd_rad
  Bus Selector5 : BusSelector  OutputSignals=Reset
  Discrete-Time Integrator1 : DiscreteIntegrator  IntegratorMethod=Integration: Trapezoidal  ExternalReset=level  SampleTime=dt
  Get_NCV : Subsystem
  Kc : Gain  Gain=kcb
  Kf : Gain  Gain=kfb
  Ki : Gain  Gain=kib
  Kp : Gain  Gain=kpb
  Sum1 : Sum  Inputs=+++
  Sum2 : Sum  Inputs=|+-
  Sum3 : Sum  Inputs=|+-
  n1 : Gain  Gain=-1
  NCVdt : Outport
  wires:
  Bus Selector3/1 -> Sum2/1, Kf/1  "<BETAcmd_rad>"
  Sum2/1 -> Ki/1, Kp/1
  CMD/1 -> Bus Selector3/1, Bus Selector5/1
  Bus Selector1/1 -> Sum2/2  "<BETA_rad>"
  Sum1/1 -> n1/1
  n1/1 -> Sum3/1
  Sum3/1 -> Kc/1
  Kc/1 -> NCVdt/1
  Kf/1 -> Sum1/1
  Kp/1 -> Sum1/3
  Bus Selector5/1 -> Discrete-Time Integrator1/2  "<Reset>"
  Ki/1 -> Discrete-Time Integrator1/1
  Discrete-Time Integrator1/1 -> Sum1/2
  Get_NCV/1(NCV) -> Sum3/2
  INPUT/1 -> Bus Selector1/1, Get_NCV/1(Input)

== system admire_sim_NDI/NDI_CLAW/DynamicInversionControl/Unom/Get_Unom ==
  Uact : Inport
  Uz : Inport  Port=2
  Constant3 : Constant  Value=4  OutDataTypeStr=int8
  Multiport Switch : MultiPortSwitch  Inputs=4
  Utrim : Constant  Value=u0new
  Uzero : Constant  Value=zeros(16,1)
  Unom : Outport
  wires:
  Multiport Switch/1 -> Unom/1  "Unom"
  Constant3/1 -> Multiport Switch/1
  Uzero/1 -> Multiport Switch/2
  Utrim/1 -> Multiport Switch/3
  Uz/1 -> Multiport Switch/4
  Uact/1 -> Multiport Switch/5

== system admire_sim_NDI/NDI_CLAW/MissionManager/WaypointNavigation/ChangeWptNumber ==
  INPUT : Inport
  WNz : Inport  Port=2
  Bus Selector1 : BusSelector  OutputSignals=X_m,Y_m  OutputAsBus=on
  Bus Selector4 : BusSelector  OutputSignals=Xcmd,Ycmd  OutputAsBus=on
  Dot Product : DotProduct  InputSameDT=on  OutDataTypeStr=Inherit: Inherit via internal rule
  Gain1 : Gain  Gain=16
  GetTurnDist : Subsystem
  Product : Product  RndMeth=Zero
  Relational Operator : RelationalOperator  Operator=<=  OutDataTypeStr=boolean
  Sum : Sum  Inputs=|+-
  Sum1 : Sum  Inputs=|++
  NextPt : Outport
  PHImax_rad : Outport  Port=2
  wires:
  WNz/1 -> Bus Selector4/1, GetTurnDist/2(WNz)
  INPUT/1 -> Bus Selector1/1, GetTurnDist/1(INPUT)
  Bus Selector4/1 -> Sum/1
  Bus Selector1/1 -> Sum/2
  Sum/1 -> Dot Product/1, Dot Product/2
  Dot Product/1 -> Relational Operator/1
  Relational Operator/1 -> NextPt/1
  GetTurnDist/2(TurnDist_m) -> Product/1, Product/2
  GetTurnDist/1(V2) -> Gain1/1
  Product/1 -> Sum1/2
  Gain1/1 -> Sum1/1
  GetTurnDist/3(PHImax_rad) -> PHImax_rad/1
  Sum1/1 -> Relational Operator/2

== system admire_sim_NDI/NDI_CLAW/MissionManager/WaypointNavigation/GetWptNumber ==
  NextPt : Inport
  Bus Creator : BusCreator  Inputs=3
  Constant{,1,3,5} (4 alike) : Constant  OutDataTypeStr=int32
  Constant2 : Constant  Value=nwpt  OutDataTypeStr=int32
  Constant4 : Constant  Value=nwpt  OutDataTypeStr=int32
  MinMax : MinMax  Inputs=2
  Relational Operator : RelationalOperator  OutDataTypeStr=boolean
  Sum : Sum  Inputs=|++
  Sum1 : Sum  Inputs=-+|
  Sum2 : Sum  Inputs=|++
  Switch : Switch  Criteria=u2 > Threshold  OutDataTypeStr=int32
  Switch1 : Switch  Criteria=u2 > Threshold  OutDataTypeStr=int32
  Unit Delay : UnitDelay  SampleTime=dt
  Out1 : Outport
  wires:
  Switch/1 -> Switch1/3, Relational Operator/1  "npt"
  Unit Delay/1 -> Switch/3, Sum/2
  Sum/1 -> Switch/1
  Constant/1 -> Sum/1
  Constant2/1 -> Relational Operator/2
  NextPt/1 -> Switch/2
  Bus Creator/1 -> Out1/1
  Constant3/1 -> Sum1/1
  Sum1/1 -> Bus Creator/1  "nptm1"
  MinMax/1 -> Bus Creator/3  "nptp1"
  Constant4/1 -> MinMax/1
  Sum2/1 -> MinMax/2
  Constant1/1 -> Sum2/2
  Relational Operator/1 -> Switch1/2
  Constant5/1 -> Switch1/1
  Switch1/1 -> Sum1/2, Bus Creator/2, Unit Delay/1, Sum2/1  "npt"

== system admire_sim_NDI/NDI_CLAW/DynamicInversionControl/AERO_OBM/AeroLimits/Get_Umax ==
  Mach : Inport
  Carnard_max : Lookup  InputValues=M_vec  Table=Canard_max  LookUpMeth=Use Input Above
  ConstantMax : Constant  Value=[LG_max TSS_max DTY_max DTZ_max UD_max VD_max WD_max PD_max]
  Elevon_max : Lookup  InputValues=M_vec  Table=Elevon_max  LookUpMeth=Use Input Above
  LEF_max : Lookup  InputValues=M_vec  Table=LEF_max  LookUpMeth=Use Input Above
  Mux2 : Mux  Inputs=9
  Rudder_max : Lookup  InputValues=M_vec  Table=Rudder_max  LookUpMeth=Use Input Above
  Umax : Outport
  wires:
  Carnard_max/1 -> Mux2/1, Mux2/2
  Elevon_max/1 -> Mux2/6, Mux2/5, Mux2/4, Mux2/3
  Rudder_max/1 -> Mux2/7
  LEF_max/1 -> Mux2/8
  Mux2/1 -> Umax/1  "Umax"
  Mach/1 -> LEF_max/1, Rudder_max/1, Elevon_max/1, Carnard_max/1
  ConstantMax/1 -> Mux2/9

== system admire_sim_NDI/NDI_CLAW/DynamicInversionControl/AERO_OBM/AeroLimits/Get_Umin ==
  Mach : Inport
  Carnard_min : Lookup  InputValues=M_vec  Table=Canard_min  LookUpMeth=Use Input Above
  ConstantMin : Constant  Value=[LG_min TSS_min DTY_min DTZ_min UD_min VD_min WD_min PD_min]
  Elevon_min : Lookup  InputValues=M_vec  Table=Elevon_min  LookUpMeth=Use Input Above
  LEF_min : Lookup  InputValues=M_vec  Table=LEF_min  LookUpMeth=Use Input Above
  Mux1 : Mux  Inputs=9
  Rudder_min : Lookup  InputValues=M_vec  Table=Rudder_min  LookUpMeth=Use Input Above
  Umin : Outport
  wires:
  Carnard_min/1 -> Mux1/2, Mux1/1
  Elevon_min/1 -> Mux1/3, Mux1/4, Mux1/6, Mux1/5
  Rudder_min/1 -> Mux1/7
  LEF_min/1 -> Mux1/8
  Mux1/1 -> Umin/1  "Umin"
  Mach/1 -> LEF_min/1, Rudder_min/1, Elevon_min/1, Carnard_min/1
  ConstantMin/1 -> Mux1/9

== system admire_sim_NDI/NDI_CLAW/DynamicInversionControl/AERO_OBM/NonLinearOBM/Get_B_Aero ==
  Sensors : Inport
  u0 : Inport  Port=2
  uz : Inport  Port=3
  Constant : Constant  OutDataTypeStr=int32
  Constant2 : Constant  OutDataTypeStr=int32
  Constant3 : Constant  Value=du
  Dimensions : Subsystem
  Gain7 : Gain  Gain=CC  Multiplication=Matrix(K*u)
  Get_CVdt : Subsystem
  Matrix Concatenate : Concatenate  NumInputs=14  Mode=Multidimensional array  ConcatenateDimension=2
  OneColPerFrame : Subsystem
  Product2 : Product  Multiplication=Matrix(*)  RndMeth=Zero
  Rate Transition : RateTransition  X0=CB(:,1:7)  OutPortSampleTime=dt
  Sum : Sum  Inputs=|++
  Sum1 : Sum  Inputs=|++  OutDataTypeStr=int32
  Switch : Switch  Criteria=u2 > Threshold  Threshold=7
  Unit Delay : UnitDelay  SampleTime=dt
  Unit Delay2 : UnitDelay  InitialCondition=CB(:,1:7)  SampleTime=dt
  CVdt : Outport
  B : Outport  Port=2
  wires:
  u0/1 -> Matrix Concatenate/13, Matrix Concatenate/14, Matrix Concatenate/12, Matrix Concatenate/11, Matrix Concatenate/10, Matrix Concatenate/9, Matrix Concatenate/8, Matrix Concatenate/7, Matrix Concatenate/6, Matrix Concatenate/5, Matrix Concatenate/4, Matrix Concatenate/3, Matrix Concatenate/2, Dimensions/1(In1), Matrix Concatenate/1
  Matrix Concatenate/1 -> Sum/1
  Constant3/1 -> Sum/2
  Product2/1 -> Gain7/1
  Gain7/1 -> B/1
  Dimensions/1(Out1) -> Product2/1, Get_CVdt/1(Dim)
  Sensors/1 -> Get_CVdt/2(Sensors)
  Get_CVdt/1(CVdt) -> CVdt/1
  Sum/1 -> OneColPerFrame/1(In1)
  Constant/1 -> Sum1/1
  Unit Delay/1 -> Sum1/2
  Sum1/1 -> Switch/2, Switch/3
  Constant2/1 -> Switch/1
  Switch/1 -> OneColPerFrame/2(In2), Unit Delay/1
  uz/1 -> Get_CVdt/3(uz)
  OneColPerFrame/1(Out1) -> Rate Transition/1
  Rate Transition/1 -> Unit Delay2/1, Product2/2
  Unit Delay2/1 -> OneColPerFrame/3(Bz)

== system admire_sim_NDI/NDI_CLAW/DynamicInversionControl/AERO_OBM/NonLinearOBM/Get_u0 ==
  INPUT : Inport
  uz : Inport  Port=2
  Bus Selector : BusSelector  OutputSignals=Unom
  Bus Selector1 : BusSelector  OutputSignals=X_states
  Constant1 : Constant  Value=[zeros(1,6) 0.3]
  Mux : Mux
  Selector : Selector  InputPortWidth=28  Indices=[1:6 12]
  Selector1 : Selector  InputPortWidth=28  Indices=[19]
  Selector2 : Selector  InputPortWidth=16  Indices=[1:8 10 9 11 12]
  u0 : Outport
  wires:
  Selector/1 -> Mux/2
  Constant1/1 -> Mux/3
  Selector1/1 -> Mux/4
  Selector2/1 -> Mux/1
  Bus Selector1/1 -> Selector/1, Selector1/1  "<X_states>"
  Bus Selector/1 -> Selector2/1  "<Unom>"
  uz/1 -> Bus Selector/1
  INPUT/1 -> Bus Selector1/1
  Mux/1 -> u0/1

== system admire_sim_NDI/NDI_CLAW/DynamicInversionControl/ControlAllocation/GetU/CGI_4 ==
  In1 : Inport
  Action Port : ActionPort  ActionType=elseif
  MATLAB Fcn : MATLABFcn  MATLABFcn=CGIwrap(u)
  Out1 : Outport
  wires:
  MATLAB Fcn/1 -> Out1/1
  In1/1 -> MATLAB Fcn/1

== system admire_sim_NDI/NDI_CLAW/DynamicInversionControl/ControlAllocation/GetU/DirectAllocation_3 ==
  In1 : Inport
  Action Port : ActionPort  ActionType=elseif
  Bus Selector : BusSelector  OutputSignals=CVdt_des
  Bus Selector1 : BusSelector  OutputSignals=CB
  Bus Selector2 : BusSelector  OutputSignals=INDX
  Bus Selector3 : BusSelector  OutputSignals=Umin,Umax
  Constant1 : Constant  Value=0
  Constant2 : Constant  Value=[0;0]
  MATLAB Fcn : MATLABFcn  MATLABFcn=DAwrap(u)
  Math Function1 : Math  Operator=transpose  SaturateOnIntegerOverflow=on
  Math Function2 : Math  Operator=transpose  SaturateOnIntegerOverflow=on
  Math Function3 : Math  Operator=transpose  SaturateOnIntegerOverflow=on
  Matrix Concatenate : Concatenate  Mode=Multidimensional array  ConcatenateDimension=2
  Matrix Concatenate1 : Concatenate  NumInputs=3  Mode=Multidimensional array
  Matrix Concatenate2 : Concatenate  Mode=Multidimensional array  ConcatenateDimension=2
  Matrix Concatenate3 : Concatenate  Mode=Multidimensional array
  Matrix Concatenate4 : Concatenate  Mode=Multidimensional array  ConcatenateDimension=2
  Signal Specification : SignalSpecification  Dimensions=[3 1]
  Signal Specification1 : SignalSpecification  Dimensions=[NumU 1]
  Signal Specification2 : SignalSpecification  Dimensions=[NumU 1]
  Signal Specification3 : SignalSpecification  Dimensions=[NumU 1]
  Out1 : Outport
  wires:
  MATLAB Fcn/1 -> Out1/1
  In1/1 -> Bus Selector/1, Bus Selector1/1, Bus Selector2/1, Bus Selector3/1
  Bus Selector/1 -> Signal Specification/1  "<CVdt_des>"
  Bus Selector1/1 -> Matrix Concatenate/1  "<CB>"
  Matrix Concatenate/1 -> Matrix Concatenate1/1
  Matrix Concatenate4/1 -> Matrix Concatenate1/2
  Signal Specification/1 -> Matrix Concatenate/2
  Bus Selector3/1 -> Signal Specification1/1  "<Umin>"
  Bus Selector3/2 -> Signal Specification2/1  "<Umax>"
  Math Function1/1 -> Matrix Concatenate3/1
  Math Function2/1 -> Matrix Concatenate3/2
  Matrix Concatenate3/1 -> Matrix Concatenate4/1
  Constant2/1 -> Matrix Concatenate4/2
  Signal Specification1/1 -> Math Function1/1
  Signal Specification2/1 -> Math Function2/1
  Constant1/1 -> Matrix Concatenate2/2
  Bus Selector2/1 -> Signal Specification3/1  "<INDX>"
  Signal Specification3/1 -> Math Function3/1
  Matrix Concatenate2/1 -> Matrix Concatenate1/3
  Math Function3/1 -> Matrix Concatenate2/1
  Matrix Concatenate1/1 -> MATLAB Fcn/1

== system admire_sim_NDI/NDI_CLAW/DynamicInversionControl/ControlAllocation/GetU/LP_6 ==
  In1 : Inport
  Action Port : ActionPort  ActionType=else
  MATLAB Fcn : MATLABFcn  MATLABFcn=LPwrap(u)
  Out1 : Outport
  wires:
  MATLAB Fcn/1 -> Out1/1
  In1/1 -> MATLAB Fcn/1
